simulink model "local_mins"  (R2022b)
settings: Solver=VariableStepDiscrete  StartTime=0.0  StopTime=100  RelTol=1e-3  EnableMultiTasking=on
settings Model: Creator=jrivitus  LastModifiedBy=bensweet
settings SolverCC: AlgebraicLoopSolver=TrustRegion
settings DataIOCC: LimitDataPoints=on  SaveFormat=Array  ReturnWorkspaceOutputs=off
settings OptimizationCC: ExpressionDepthLimit=2147483647  LifeSpan=inf
settings DebuggingCC: UnconnectedInputMsg=warning  UnconnectedOutputMsg=warning  UnconnectedLineMsg=warning  PregeneratedLibrarySubsystemCodeDiagnostic=none  SFMachineParentedDataDiag=warning
settings HardwareCC: ProdBitPerPointer=32  ProdBitPerSizeT=32  ProdBitPerPtrDiffT=32  ProdLargestAtomicFloat=None  ProdIntDivRoundTo=Undefined  ProdEndianess=Unspecified  ProdWordSize=32  ProdHWDeviceType=32-bit Generic
settings ModelReferenceCC: EnableRefExpFcnMdlSchedulingChecks=on  PropagateSignalLabelsOutOfModel=off
settings SFSimCC: SimUseLocalCustomCode=off
settings RTWCC: RTWUseLocalCustomCode=off  DLArmComputeVersion=19.05
settings CodeAppCC: StateflowObjectComments=on
settings GRTTargetCC: TargetLangStandard=C89/C90 (ANSI)
settings ConfigComp: CovMetricSettings=dw  CovSaveCumulativeToWorkspaceVar=on  CovSaveSingleToWorkspaceVar=on  CovExternalEMLEnable=off  CovSFcnEnable=off

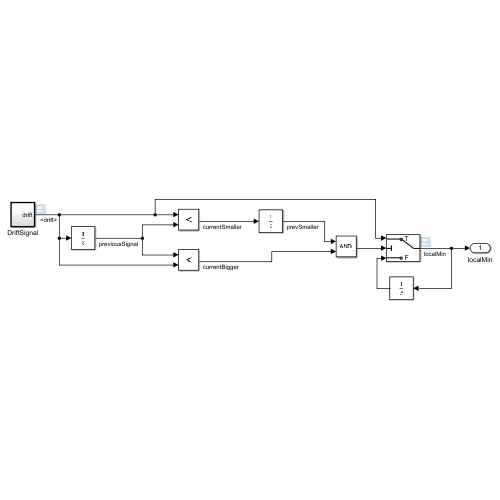
[thumbnail: Simulink's stored preview of the top-level diagram]
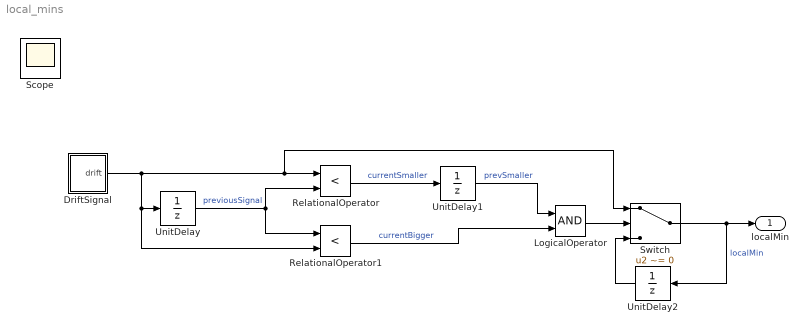
== system local_mins ==
  DriftSignal : Subsystem  TreatAsAtomicUnit=on  SystemSampleTime=1
  LogicalOperator : Logic  AllPortsSameDT=off  OutDataTypeStr=boolean
  RelationalOperator : RelationalOperator  Operator=<  OutDataTypeStr=boolean  InputSameDT=off
  RelationalOperator1 : RelationalOperator  Operator=<  OutDataTypeStr=boolean  InputSameDT=off
  Switch : Switch  Criteria=u2 ~= 0  SaturateOnIntegerOverflow=off  InputSameDT=off
  UnitDelay : UnitDelay  SampleTime=-1  HasFrameUpgradeWarning=on
  UnitDelay1 : UnitDelay  HasFrameUpgradeWarning=on
  UnitDelay2 : UnitDelay  HasFrameUpgradeWarning=on
  localMin : Outport  VectorParamsAs1DForOutWhenUnconnected=off
  Scope : Scope
  wires:
  UnitDelay1/1 -> LogicalOperator/1  "prevSmaller"
  RelationalOperator/1 -> UnitDelay1/1  "currentSmaller"
  UnitDelay/1 -> RelationalOperator/2, RelationalOperator1/1  "previousSignal"
  RelationalOperator1/1 -> LogicalOperator/2  "currentBigger"
  LogicalOperator/1 -> Switch/2
  DriftSignal/1(drift) -> RelationalOperator1/2, UnitDelay/1, RelationalOperator/1, Switch/1
  Switch/1 -> localMin/1, UnitDelay2/1  "localMin"
  UnitDelay2/1 -> Switch/3

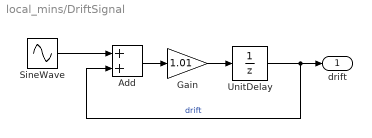
== system local_mins/DriftSignal ==
  Add : Sum
  Gain : Gain  Gain=1.01
  SineWave : Sin  Frequency=2*pi/10.3  SampleTime=1
  UnitDelay : UnitDelay  HasFrameUpgradeWarning=on
  drift : Outport  VectorParamsAs1DForOutWhenUnconnected=off
  wires:
  UnitDelay/1 -> drift/1, Add/2  "drift"
  SineWave/1 -> Add/1
  Add/1 -> Gain/1
  Gain/1 -> UnitDelay/1
